simulink model "scara"  (R2018b)
settings: Solver=VariableStepAuto  StartTime=0.0  StopTime=inf  RelTol=1e-3
libraries: simulink x2
settings Model: Creator=Bartlomiej Mroz  LastModifiedBy=Bartlomiej Mroz

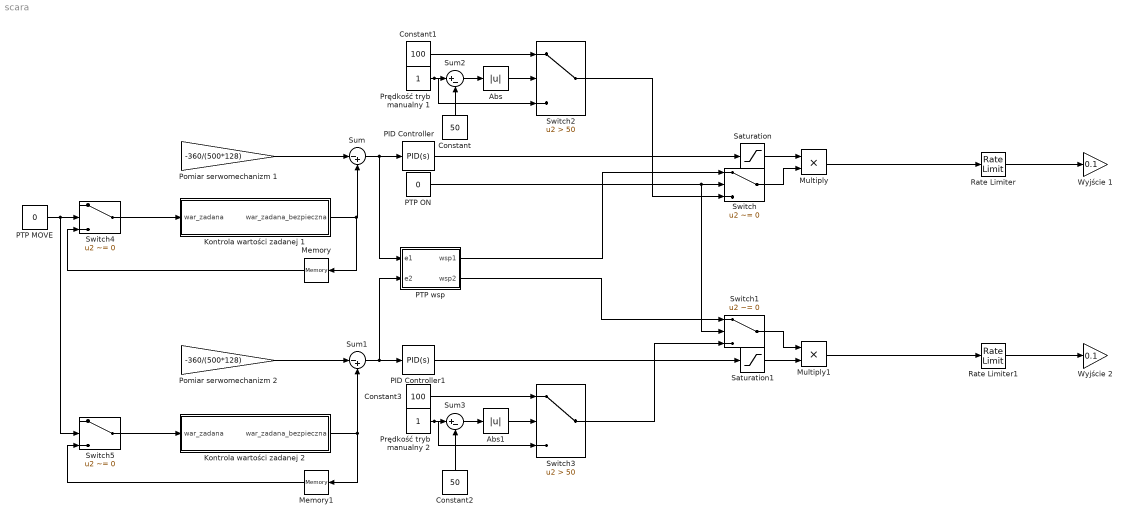
== system scara ==
  Abs : Abs
  Abs1 : Abs
  Constant : Constant  Value=50
  Constant1 : Constant  Value=100
  Constant2 : Constant  Value=50
  Constant3 : Constant  Value=100
  "Kontrola wartości zadanej 1 " : Subsystem
  Kontrola wartości zadanej 2 : Subsystem
  Memory : Memory
  Memory1 : Memory
  Multiply : Product
  Multiply1 : Product
  PID Controller : simulink/Continuous/PID Controller  Controller=PID  Form=Parallel  TimeDomain=Continuous-time  SampleTime=-1  IntegratorMethod=Forward Euler  FilterMethod=Forward Euler  ControllerParametersSource=internal  P=0.2  I=0  D=0  UseFilter=on  N=100  TunerSelectOption=Transfer Function Based (PID Tuner App)  InitialConditionSource=internal  InitialConditionForIntegrator=0  InitialConditionForFilter=0  DifferentiatorICPrevScaledInput=0  ExternalReset=none  TrackingMode=off  Kt=1  LimitOutput=off  UpperSaturationLimit=inf  LowerSaturationLimit=-inf  LinearizeAsGain=on  AntiWindupMode=none  Kb=1  POutMin=[]  POutMax=[]  IOutMin=[]  IOutMax=[]  DOutMin=[]  DOutMax=[]  NOutMin=[]  NOutMax=[]  SumOutMin=[]  SumOutMax=[]  SaturationOutMin=[]  SaturationOutMax=[]  PParamMin=[]  PParamMax=[]  IParamMin=[]  IParamMax=[]  DParamMin=[]  DParamMax=[]  NParamMin=[]  NParamMax=[]  KbParamMin=[]  KbParamMax=[]  KtParamMin=[]  KtParamMax=[]  KbOutMin=[]  KbOutMax=[]  KtOutMin=[]  KtOutMax=[]  IntegratorOutMin=[]  IntegratorOutMax=[]  FilterOutMin=[]  FilterOutMax=[]  SumI1OutMin=[]  SumI1OutMax=[]  SumI2OutMin=[]  SumI2OutMax=[]  SumI3OutMin=[]  SumI3OutMax=[]  SumI4OutMin=[]  SumI4OutMax=[]  SumDOutMin=[]  SumDOutMax=[]  DifferentiatorOutMin=[]  DifferentiatorOutMax=[]  FilterDiffOutCoefMin=[]  FilterDiffOutCoefMax=[]  ReciprocalOutMin=[]  ReciprocalOutMax=[]  SumDenOutMin=[]  SumDenOutMax=[]  SumNumOutMin=[]  SumNumOutMax=[]  DivideOutMin=[]  DivideOutMax=[]  IntegratorContinuousStateAttributes=''  IntegratorStateMustResolveToSignalObject=off  IntegratorRTWStateStorageClass=Auto  FilterContinuousStateAttributes=''  FilterStateMustResolveToSignalObject=off  FilterRTWStateStorageClass=Auto  ParallelPVariant=InternalParameters  IdealPVariant=Disabled  IVariant=InternalParameters  DVariant=InternalParameters  IntegratorVariant=Continuous  SatVariant=Disabled  AWVariant=Passthrough  PCopyVariant=Disabled  TRVariant=Disabled  FdbkBlocksVariant=Forward  IdealPFdbkVariant=Disabled  SatFdbkVariant=Disabled  DerivativeFilterVariant=ContFilter  NVariant=InternalParameters  NCopyVariant=Disabled  FilterICVariant=InternalICsFilter  IntegratorICVariant=InternalICs  ExternalResetVariant=Disabled  TRSumVariant=Passthrough  SumFdbkVariant=Disabled  SumVariant=Sum_PID
  PID Controller1 : simulink/Continuous/PID Controller  Controller=PID  Form=Parallel  TimeDomain=Continuous-time  SampleTime=-1  IntegratorMethod=Forward Euler  FilterMethod=Forward Euler  ControllerParametersSource=internal  P=0.2  I=0  D=0  UseFilter=on  N=100  TunerSelectOption=Transfer Function Based (PID Tuner App)  InitialConditionSource=internal  InitialConditionForIntegrator=0  InitialConditionForFilter=0  DifferentiatorICPrevScaledInput=0  ExternalReset=none  TrackingMode=off  Kt=1  LimitOutput=off  UpperSaturationLimit=inf  LowerSaturationLimit=-inf  LinearizeAsGain=on  AntiWindupMode=none  Kb=1  POutMin=[]  POutMax=[]  IOutMin=[]  IOutMax=[]  DOutMin=[]  DOutMax=[]  NOutMin=[]  NOutMax=[]  SumOutMin=[]  SumOutMax=[]  SaturationOutMin=[]  SaturationOutMax=[]  PParamMin=[]  PParamMax=[]  IParamMin=[]  IParamMax=[]  DParamMin=[]  DParamMax=[]  NParamMin=[]  NParamMax=[]  KbParamMin=[]  KbParamMax=[]  KtParamMin=[]  KtParamMax=[]  KbOutMin=[]  KbOutMax=[]  KtOutMin=[]  KtOutMax=[]  IntegratorOutMin=[]  IntegratorOutMax=[]  FilterOutMin=[]  FilterOutMax=[]  SumI1OutMin=[]  SumI1OutMax=[]  SumI2OutMin=[]  SumI2OutMax=[]  SumI3OutMin=[]  SumI3OutMax=[]  SumI4OutMin=[]  SumI4OutMax=[]  SumDOutMin=[]  SumDOutMax=[]  DifferentiatorOutMin=[]  DifferentiatorOutMax=[]  FilterDiffOutCoefMin=[]  FilterDiffOutCoefMax=[]  ReciprocalOutMin=[]  ReciprocalOutMax=[]  SumDenOutMin=[]  SumDenOutMax=[]  SumNumOutMin=[]  SumNumOutMax=[]  DivideOutMin=[]  DivideOutMax=[]  IntegratorContinuousStateAttributes=''  IntegratorStateMustResolveToSignalObject=off  IntegratorRTWStateStorageClass=Auto  FilterContinuousStateAttributes=''  FilterStateMustResolveToSignalObject=off  FilterRTWStateStorageClass=Auto  ParallelPVariant=InternalParameters  IdealPVariant=Disabled  IVariant=InternalParameters  DVariant=InternalParameters  IntegratorVariant=Continuous  SatVariant=Disabled  AWVariant=Passthrough  PCopyVariant=Disabled  TRVariant=Disabled  FdbkBlocksVariant=Forward  IdealPFdbkVariant=Disabled  SatFdbkVariant=Disabled  DerivativeFilterVariant=ContFilter  NVariant=InternalParameters  NCopyVariant=Disabled  FilterICVariant=InternalICsFilter  IntegratorICVariant=InternalICs  ExternalResetVariant=Disabled  TRSumVariant=Passthrough  SumFdbkVariant=Disabled  SumVariant=Sum_PID
  PTP MOVE : Constant  Value=0
  "PTP ON " : Constant  Value=0
  "PTP wsp " : MATLAB Function  TreatAsAtomicUnit=on
  Pomiar serwomechanizm 1 : Gain  Gain=-360/(500*128)
  Pomiar serwomechanizm 2 : Gain  Gain=-360/(500*128)
  Prędkość tryb manualny 1 : Constant
  Prędkość tryb manualny 2 : Constant
  Rate Limiter : RateLimiter  RisingSlewLimit=50  FallingSlewLimit=-50  SampleTimeMode=inherited
  Rate Limiter1 : RateLimiter  RisingSlewLimit=50  FallingSlewLimit=-50  SampleTimeMode=inherited
  Saturation : Saturate  UpperLimit=3  LowerLimit=-3
  Saturation1 : Saturate  UpperLimit=3  LowerLimit=-3
  Sum : Sum  Inputs=|-+
  Sum1 : Sum  Inputs=|-+
  Sum2 : Sum  Inputs=|+-
  Sum3 : Sum  Inputs=|+-
  Switch{,1,4..5} (4 alike) : Switch  Criteria=u2 ~= 0
  Switch2 : Switch  Criteria=u2 > Threshold  Threshold=50
  Switch3 : Switch  Criteria=u2 > Threshold  Threshold=50
  Wyjście 1 : Gain  Gain=0.1
  Wyjście 2 : Gain  Gain=0.1
  wires:
  Pomiar serwomechanizm 1/1 -> Sum/1
  "Kontrola wartości zadanej 1 "/1(war_zadana_bezpieczna) -> Memory/1, Sum/2
  Kontrola wartości zadanej 2/1(war_zadana_bezpieczna) -> Memory1/1, Sum1/2
  Pomiar serwomechanizm 2/1 -> Sum1/1
  Sum/1 -> "PTP wsp "/1(e1), PID Controller/1
  Sum1/1 -> "PTP wsp "/2(e2), PID Controller1/1
  PID Controller/1 -> Saturation/1
  PID Controller1/1 -> Saturation1/1
  Rate Limiter/1 -> Wyjście 1/1
  Rate Limiter1/1 -> Wyjście 2/1
  "PTP ON "/1 -> Switch1/2, Switch/2
  Saturation/1 -> Multiply/1
  Saturation1/1 -> Multiply1/2
  Multiply1/1 -> Rate Limiter1/1
  Multiply/1 -> Rate Limiter/1
  Switch/1 -> Multiply/2
  Switch1/1 -> Multiply1/1
  "PTP wsp "/1(wsp1) -> Switch/1
  "PTP wsp "/2(wsp2) -> Switch1/1
  Prędkość tryb manualny 1/1 -> Switch2/3, Sum2/1
  Constant/1 -> Sum2/2
  Sum2/1 -> Abs/1
  Abs/1 -> Switch2/2
  Constant1/1 -> Switch2/1
  Constant3/1 -> Switch3/1
  Abs1/1 -> Switch3/2
  Sum3/1 -> Abs1/1
  Constant2/1 -> Sum3/2
  Prędkość tryb manualny 2/1 -> Sum3/1, Switch3/3
  Switch3/1 -> Switch1/3
  Switch2/1 -> Switch/3
  PTP MOVE/1 -> Switch5/2, Switch4/2
  Switch4/1 -> "Kontrola wartości zadanej 1 "/1(war_zadana)
  Switch5/1 -> Kontrola wartości zadanej 2/1(war_zadana)
  Memory/1 -> Switch4/3
  Memory1/1 -> Switch5/3

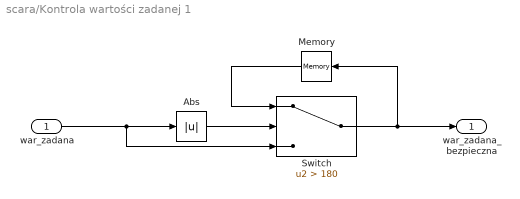
== system scara/Kontrola wartości zadanej 1  ==
  war_zadana : Inport
  Abs : Abs
  Memory : Memory
  Switch : Switch  Criteria=u2 > Threshold  Threshold=180
  war_zadana_bezpieczna : Outport
  wires:
  war_zadana/1 -> Switch/3, Abs/1
  Abs/1 -> Switch/2
  Switch/1 -> Memory/1, war_zadana_bezpieczna/1
  Memory/1 -> Switch/1

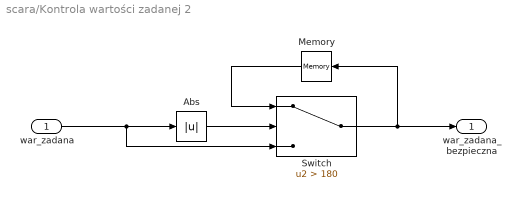
== system scara/Kontrola wartości zadanej 2 ==
  war_zadana : Inport
  Abs : Abs
  Memory : Memory
  Switch : Switch  Criteria=u2 > Threshold  Threshold=180
  war_zadana_bezpieczna : Outport
  wires:
  Memory/1 -> Switch/1
  Switch/1 -> war_zadana_bezpieczna/1, Memory/1
  Abs/1 -> Switch/2
  war_zadana/1 -> Abs/1, Switch/3

== matlab function scara/PTP wsp  ==
  data: e1 input; wsp1 output; e2 input; wsp2 output
function [wsp1,wsp2] = fcn(e1,e2)
denum = max(e1,e2);
wsp1 = e1/denum;
wsp2 = e2/denum;
